simulink model "pidmodel1"  (R2013a)
settings: Solver=ode45  StartTime=0.0  StopTime=10.0  RelTol=1e-3
values from neighbouring files (symbols this model uses):
  A = [0,0,1,0;0,0,0,1;-0,2,3.5,0;0,-3,-2,0]    [at.m]
  B = [0;0;-2;-3]    [at.m]
  C = [1,0,0,0;0,1,0,0;0,0,1,0;0,0,0,1]    [at.m]
  D = [0;0;0;0]    [at.m]
  g = 9.8    [at.m]
  Jp = 0.2    [at.m]
  Jw = 2.3    [at.m]
  Ke = 3    [at.m]
  Kt = 5    [at.m]
  L = 1.8    [at.m]
  mp = 0.9    [at.m]
  mw = 0.2    [at.m]
  n = 0.9    [at.m]
  r = 0.9    [at.m]
  Ra = 0.9    [at.m]
libraries: simulink x2
settings Model: Creator=user  LastModifiedBy=user

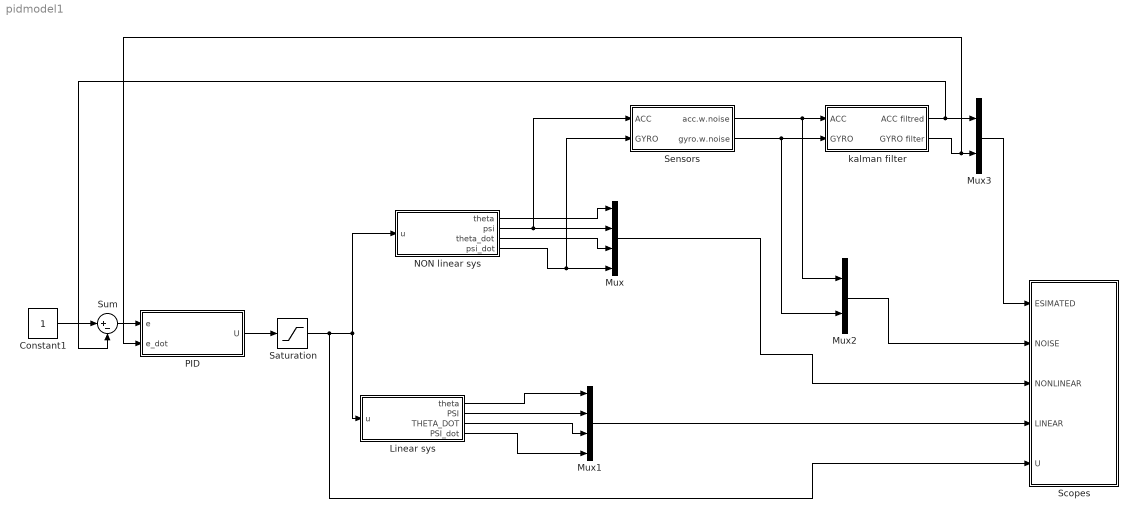
== system pidmodel1 ==
  Constant1 : Constant
  Linear sys : Subsystem
  Mux : Mux
  Mux1 : Mux
  Mux2 : Mux  Inputs=2
  Mux3 : Mux  Inputs=2
  NON linear sys : Subsystem
  "PID " : Subsystem
  Saturation : Saturate
  Scopes : Subsystem
  Sensors : Subsystem
  Sum : Sum  Inputs=|+-
  kalman filter : Subsystem
  wires:
  Sum/1 -> "PID "/1(e)
  Constant1/1 -> Sum/1
  "PID "/1(U) -> Saturation/1
  Linear sys/1(theta) -> Mux1/1
  Linear sys/2(PSI) -> Mux1/2
  Linear sys/3(THETA_DOT) -> Mux1/3
  Linear sys/4(PSI_dot) -> Mux1/4
  NON linear sys/1(theta) -> Mux/1
  NON linear sys/2(psi) -> Sensors/1(ACC), Mux/2
  NON linear sys/3(theta_dot) -> Mux/3
  NON linear sys/4(psi_dot) -> Sensors/2("GYRO "), Mux/4
  Sensors/1(acc.w.noise) -> Mux2/1, kalman filter/1(ACC)
  Sensors/2("gyro.w.noise ") -> Mux2/2, kalman filter/2(GYRO)
  Mux2/1 -> Scopes/2(NOISE)
  Mux3/1 -> Scopes/1(ESIMATED)
  Mux/1 -> Scopes/3(NONLINEAR)
  Mux1/1 -> Scopes/4(LINEAR)
  Saturation/1 -> Scopes/5(U), NON linear sys/1(u), Linear sys/1(u)
  kalman filter/1(ACC filtred) -> Sum/2, Mux3/1
  kalman filter/2(GYRO filter) -> "PID "/2(e_dot), Mux3/2

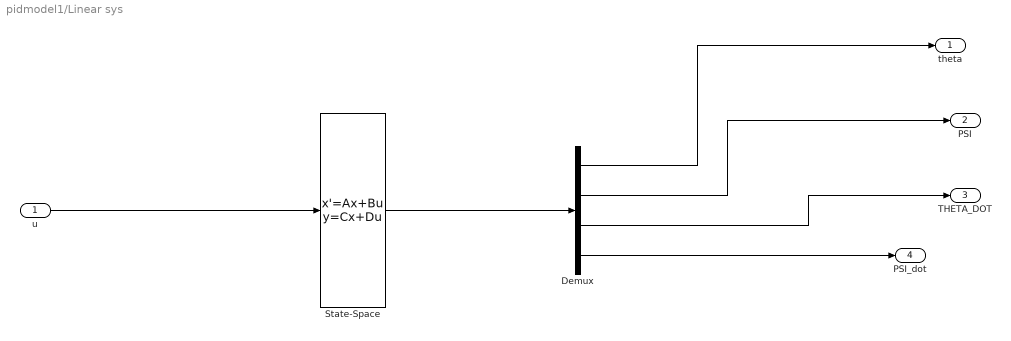
== system pidmodel1/Linear sys ==
  u : Inport
  Demux : Demux
  State-Space : StateSpace  A=A  B=B  C=C  D=D
  theta : Outport
  PSI : Outport  Port=2
  THETA_DOT : Outport  Port=3
  PSI_dot : Outport  Port=4
  wires:
  u/1 -> State-Space/1
  State-Space/1 -> Demux/1
  Demux/1 -> theta/1
  Demux/2 -> PSI/1
  Demux/3 -> THETA_DOT/1
  Demux/4 -> PSI_dot/1

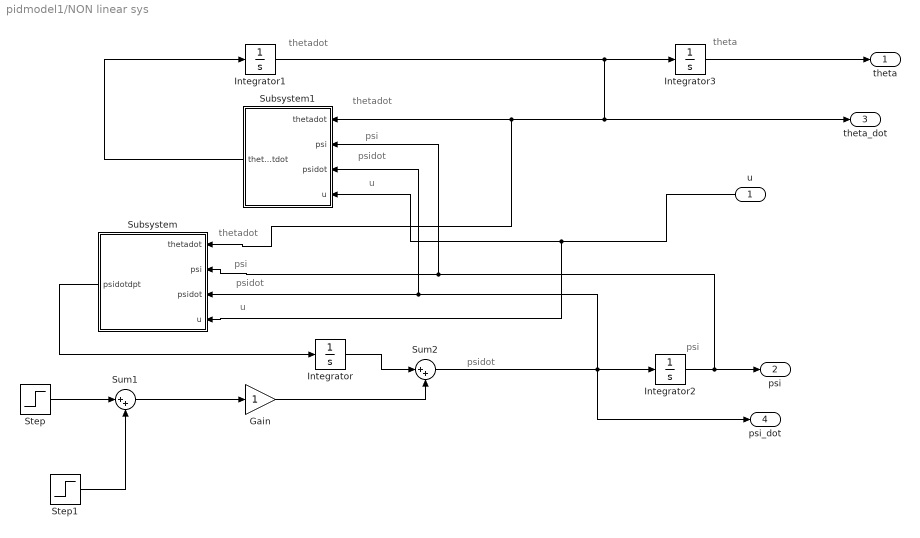
== system pidmodel1/NON linear sys ==
  note: psidot
  note: psi
  note: u
  note: theta
  note: thetadot
  note: psidot
  note: psi
  note: thetadot
  note: u
  note: psidot
  note: psi
  note: thetadot
  u : Inport
  Gain : Gain
  Integrator{,1..3} (4 alike) : Integrator
  Step : Step  SampleTime=0
  Step1 : Step  SampleTime=0
  Subsystem : Subsystem
  Subsystem1 : Subsystem
  Sum1 : Sum  Inputs=|++
  Sum2 : Sum  Inputs=|++
  theta : Outport
  psi : Outport  Port=2
  theta_dot : Outport  Port=3
  psi_dot : Outport  Port=4
  wires:
  Step/1 -> Sum1/1
  Step1/1 -> Sum1/2
  Sum1/1 -> Gain/1
  Gain/1 -> Sum2/2
  Integrator/1 -> Sum2/1
  u/1 -> Subsystem1/4(u), Subsystem/4(u)
  Sum2/1 -> psi_dot/1, Integrator2/1, Subsystem1/3(psidot), Subsystem/3(psidot)
  Integrator2/1 -> Subsystem/2(psi), Subsystem1/2(psi), psi/1
  Integrator1/1 -> Subsystem1/1(thetadot), Subsystem/1(thetadot), theta_dot/1, Integrator3/1
  Integrator3/1 -> theta/1
  Subsystem1/1(thetadotdot) -> Integrator1/1
  Subsystem/1(psidotdpt) -> Integrator/1

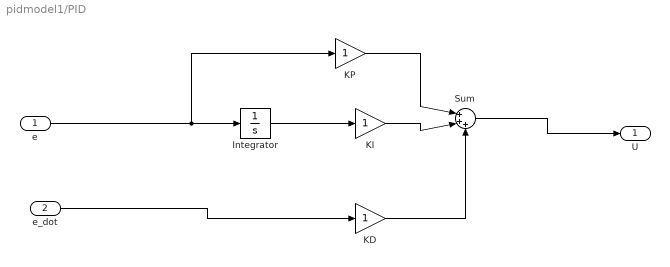
== system pidmodel1/PID  ==
  e : Inport
  e_dot : Inport  Port=2
  Integrator : Integrator
  KD : Gain
  KI : Gain
  KP : Gain
  Sum : Sum  Inputs=|+++
  U : Outport
  wires:
  e/1 -> KP/1, Integrator/1
  Integrator/1 -> KI/1
  e_dot/1 -> KD/1
  Sum/1 -> U/1
  KP/1 -> Sum/1
  KD/1 -> Sum/3
  KI/1 -> Sum/2

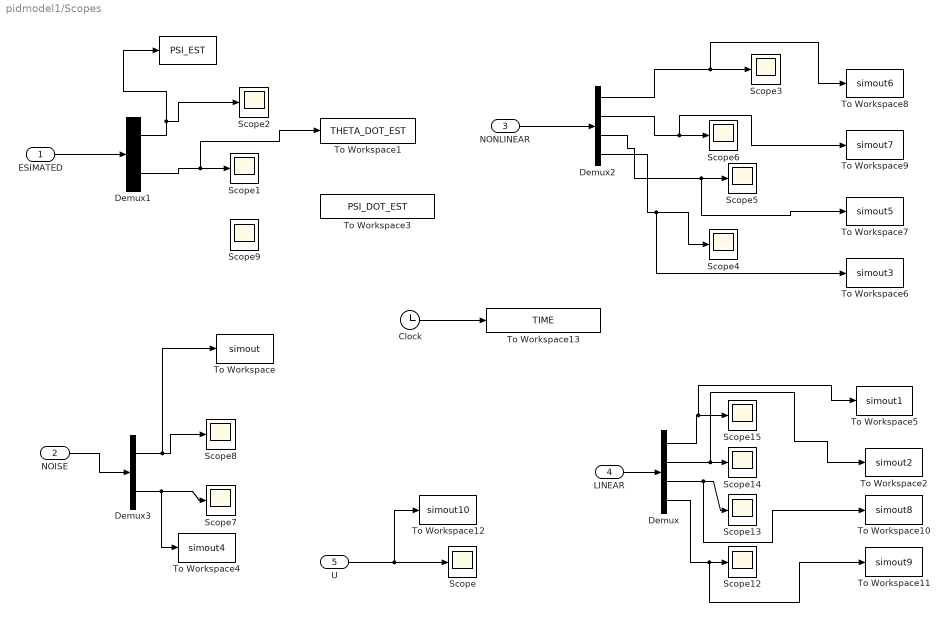
== system pidmodel1/Scopes ==
  ESIMATED : Inport
  NOISE : Inport  Port=2
  NONLINEAR : Inport  Port=3
  LINEAR : Inport  Port=4
  U : Inport  Port=5
  " " : ToWorkspace  VariableName=PSI_EST  SampleTime=-1  SaveFormat=Timeseries
  Clock : Clock
  Demux : Demux
  Demux1 : Demux  Outputs=2
  Demux2 : Demux
  Demux3 : Demux  Outputs=2
  Scope{,1..9,12..15} (14 alike) : Scope
      Scope12 settings: SaveName=ScopeData12
      Scope13 settings: SaveName=ScopeData13
      Scope14 settings: SaveName=ScopeData14
      Scope15 settings: SaveName=ScopeData15
      Scope2 settings: SaveName=ScopeData2
      Scope3 settings: SaveName=ScopeData3
      Scope4 settings: SaveName=ScopeData4
      Scope5 settings: SaveName=ScopeData5
      Scope6 settings: SaveName=ScopeData6
      Scope7 settings: SaveName=ScopeData7
      Scope8 settings: SaveName=ScopeData8
      Scope9 settings: SaveName=ScopeData9
  To Workspace : ToWorkspace  VariableName=simout  SampleTime=-1  SaveFormat=Timeseries
  To Workspace1 : ToWorkspace  VariableName=THETA_DOT_EST  SampleTime=-1  SaveFormat=Timeseries
  To Workspace10 : ToWorkspace  VariableName=simout8  SampleTime=-1  SaveFormat=Timeseries
  To Workspace11 : ToWorkspace  VariableName=simout9  SampleTime=-1  SaveFormat=Timeseries
  To Workspace12 : ToWorkspace  VariableName=simout10  SampleTime=-1  SaveFormat=Timeseries
  To Workspace13 : ToWorkspace  VariableName=TIME  SampleTime=-1  SaveFormat=Timeseries
  To Workspace2 : ToWorkspace  VariableName=simout2  SampleTime=-1  SaveFormat=Timeseries
  To Workspace3 : ToWorkspace  VariableName=PSI_DOT_EST  SampleTime=-1  SaveFormat=Timeseries
  To Workspace4 : ToWorkspace  VariableName=simout4  SampleTime=-1  SaveFormat=Timeseries
  To Workspace5 : ToWorkspace  VariableName=simout1  SampleTime=-1  SaveFormat=Timeseries
  To Workspace6 : ToWorkspace  VariableName=simout3  SampleTime=-1  SaveFormat=Timeseries
  To Workspace7 : ToWorkspace  VariableName=simout5  SampleTime=-1  SaveFormat=Timeseries
  To Workspace8 : ToWorkspace  VariableName=simout6  SampleTime=-1  SaveFormat=Timeseries
  To Workspace9 : ToWorkspace  VariableName=simout7  SampleTime=-1  SaveFormat=Timeseries
  wires:
  ESIMATED/1 -> Demux1/1
  Demux1/1 -> " "/1, Scope2/1
  Demux1/2 -> To Workspace1/1, Scope1/1
  ? -> Scope9/1, To Workspace3/1
  Demux3/2 -> To Workspace4/1, Scope7/1
  Demux3/1 -> To Workspace/1, Scope8/1
  NOISE/1 -> Demux3/1
  NONLINEAR/1 -> Demux2/1
  Demux2/1 -> To Workspace8/1, Scope3/1
  Demux2/2 -> To Workspace9/1, Scope6/1
  Demux2/4 -> To Workspace6/1, Scope4/1
  Demux2/3 -> To Workspace7/1, Scope5/1
  LINEAR/1 -> Demux/1
  Demux/1 -> To Workspace5/1, Scope15/1
  Demux/3 -> To Workspace10/1, Scope13/1
  Demux/2 -> To Workspace2/1, Scope14/1
  Demux/4 -> To Workspace11/1, Scope12/1
  U/1 -> To Workspace12/1, Scope/1
  Clock/1 -> To Workspace13/1

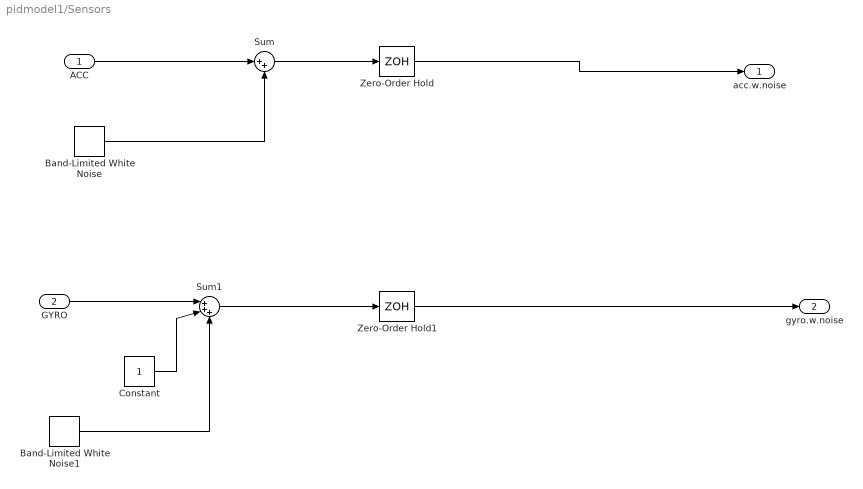
== system pidmodel1/Sensors ==
  ACC : Inport
  "GYRO " : Inport  Port=2
  Band-Limited White Noise : simulink/Sources/Band-Limited White Noise  Cov=[0.1]  Ts=0.1  seed=[23341]
  Band-Limited White Noise1 : simulink/Sources/Band-Limited White Noise  Cov=[0.1]  Ts=0.1  seed=[23341]
  Constant : Constant
  Sum : Sum  Inputs=|++
  Sum1 : Sum  Inputs=|+++
  Zero-Order Hold : ZeroOrderHold
  Zero-Order Hold1 : ZeroOrderHold
  acc.w.noise : Outport
  "gyro.w.noise " : Outport  Port=2
  wires:
  ACC/1 -> Sum/1
  Band-Limited White Noise/1 -> Sum/2
  "GYRO "/1 -> Sum1/1
  Band-Limited White Noise1/1 -> Sum1/3
  Constant/1 -> Sum1/2
  Sum1/1 -> Zero-Order Hold1/1
  Sum/1 -> Zero-Order Hold/1
  Zero-Order Hold/1 -> acc.w.noise/1
  Zero-Order Hold1/1 -> "gyro.w.noise "/1

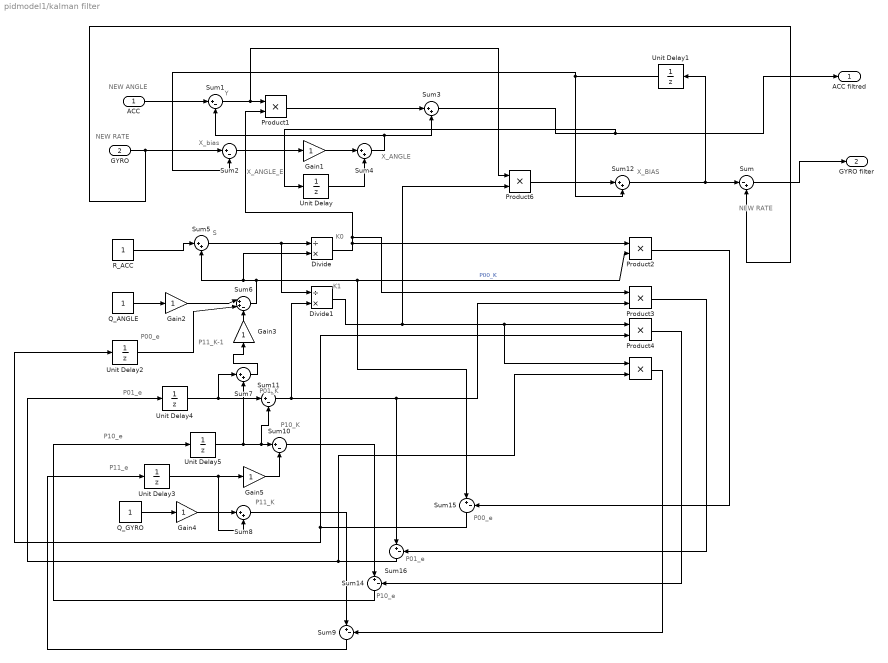
== system pidmodel1/kalman filter ==
  note: NEW RATE
  note: X_BIAS
  note: P10_e
  note: P01_e
  note: P00_e
  note: K1
  note: P01_K
  note: P01_e
  note: P11_e
  note: P10_e
  note: P10_K
  note: P11_K
  note: P00_e
  note: P11_K-1
  note: X_ANGLE_E
  note: X_ANGLE
  note: X_bias
  note: K0
  note: S
  note: Y
  note: NEW RATE
  note: NEW ANGLE
  ACC : Inport
  GYRO : Inport  Port=2
  " " : Product
  Divide : Product  Inputs=/*
  Divide1 : Product  Inputs=/*
  Gain{1..5} (5 alike) : Gain
  Product{1..4,6} (5 alike) : Product
  Q_ANGLE : Constant
  Q_GYRO : Constant
  R_ACC : Constant
  Sum : Sum  Inputs=|-+
  Sum{1..2,9..11,14..16} (8 alike) : Sum  Inputs=|+-
  Sum{3..5,7..8,12} (6 alike) : Sum  Inputs=|++
  Sum6 : Sum  Inputs=|++-
  Unit Delay{,1..5} (6 alike) : UnitDelay  SampleTime=-1
  ACC filtred : Outport
  GYRO filter : Outport  Port=2
  wires:
  ACC/1 -> Sum1/1
  Product1/1 -> Sum3/1
  Sum2/1 -> Gain1/1
  Gain1/1 -> Sum4/1
  Sum4/1 -> Sum3/2, Sum1/2
  R_ACC/1 -> Sum5/1
  Sum5/1 -> Divide1/1, Divide/1
  Q_ANGLE/1 -> Gain2/1
  Gain2/1 -> Sum6/1
  Sum6/1 -> Sum5/2, Divide/2, Sum15/1, Product2/2  "P00_K"
  Gain3/1 -> Sum6/3
  Sum7/1 -> Gain3/1
  Divide/1 -> Product2/1, Product3/1, Product1/2
  Sum3/1 -> Unit Delay/1, ACC filtred/1
  Sum15/1 -> Unit Delay2/1, Product4/2
  Q_GYRO/1 -> Gain4/1
  Gain4/1 -> Sum8/1
  Sum8/1 -> Sum9/1
  " "/1 -> Sum9/2
  Sum9/1 -> Unit Delay3/1
  Unit Delay3/1 -> Gain5/1, Sum8/2
  Gain5/1 -> Sum10/2
  Unit Delay5/1 -> Sum7/2, Sum11/2, Sum10/1
  Sum14/1 -> Unit Delay5/1
  Unit Delay4/1 -> Sum7/1, Sum11/1
  Sum11/1 -> Divide1/2, Sum16/1, Product3/2
  Divide1/1 -> Product6/2, " "/1, Product4/1
  Product2/1 -> Sum15/2
  Product3/1 -> Sum16/2
  Product4/1 -> Sum14/2
  Sum10/1 -> Sum14/1
  Sum16/1 -> " "/2, Unit Delay4/1
  Sum1/1 -> Product6/1, Product1/1
  Product6/1 -> Sum12/1
  Unit Delay1/1 -> Sum2/2, Sum12/2
  Sum12/1 -> Unit Delay1/1, Sum/1
  Sum/1 -> GYRO filter/1
  GYRO/1 -> Sum/2, Sum2/1
  Unit Delay/1 -> Sum4/2
  Unit Delay2/1 -> Sum6/2

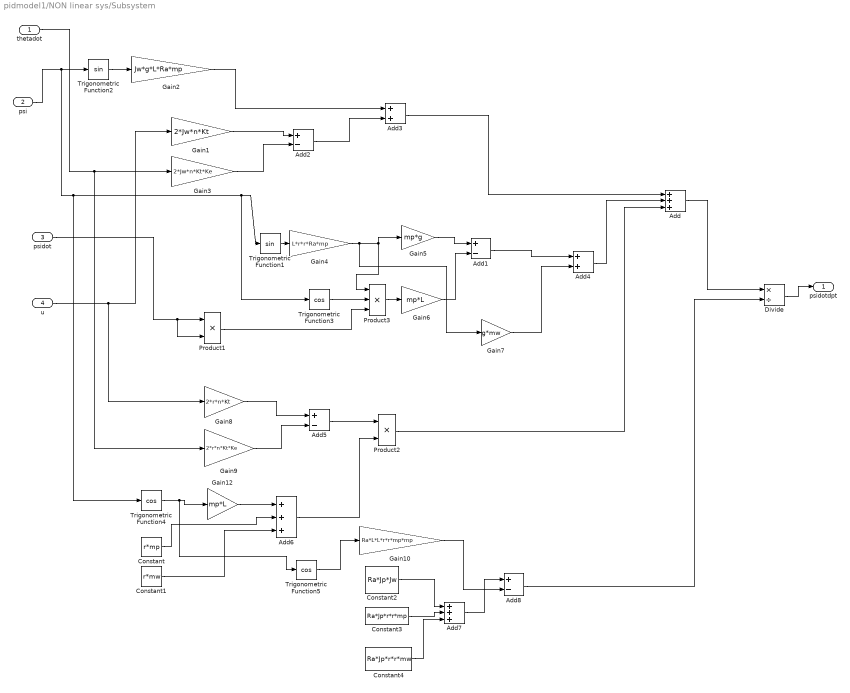
== system pidmodel1/NON linear sys/Subsystem ==
  thetadot : Inport
  psi : Inport  Port=2
  psidot : Inport  Port=3
  u : Inport  Port=4
  Add : Sum  Inputs=+++
  Add{1..2,5,8} (4 alike) : Sum  Inputs=+-
  Add3 : Sum
  Add4 : Sum
  Add6 : Sum  Inputs=+++
  Add7 : Sum  Inputs=+++
  Constant : Constant  Value=r*mp
  Constant1 : Constant  Value=r*mw
  Constant2 : Constant  Value=Ra*Jp*Jw
  Constant3 : Constant  Value=Ra*Jp*r*r*mp
  Constant4 : Constant  Value=Ra*Jp*r*r*mw
  Divide : Product  Inputs=*/
  Gain1 : Gain  Gain=2*Jw*n*Kt
  Gain10 : Gain  Gain=Ra*L*L*r*r*mp*mp
  Gain12 : Gain  Gain=mp*L
  Gain2 : Gain  Gain=Jw*g*L*Ra*mp
  Gain3 : Gain  Gain=2*Jw*n*Kt*Ke
  Gain4 : Gain  Gain=L*r*r*Ra*mp
  Gain5 : Gain  Gain=mp*g
  Gain6 : Gain  Gain=mp*L
  Gain7 : Gain  Gain=g*mw
  Gain8 : Gain  Gain=2*r*n*Kt
  Gain9 : Gain  Gain=2*r*n*Kt*Ke
  Product1 : Product
  Product2 : Product
  Product3 : Product  Inputs=3
  Trigonometric Function1 : Trigonometry
  Trigonometric Function2 : Trigonometry
  Trigonometric Function3 : Trigonometry  Operator=cos
  Trigonometric Function4 : Trigonometry  Operator=cos
  Trigonometric Function5 : Trigonometry  Operator=cos
  psidotdpt : Outport
  wires:
  Gain2/1 -> Add3/1
  u/1 -> Gain8/1, Gain1/1
  Gain1/1 -> Add2/1
  thetadot/1 -> Gain9/1, Gain3/1
  Gain3/1 -> Add2/2
  Add2/1 -> Add3/2
  psi/1 -> Trigonometric Function4/1, Trigonometric Function3/1, Trigonometric Function1/1, Trigonometric Function2/1
  Trigonometric Function2/1 -> Gain2/1
  Add3/1 -> Add/1
  Trigonometric Function1/1 -> Gain4/1
  psidot/1 -> Product1/2, Product1/1
  Gain6/1 -> Add1/2
  Product1/1 -> Product3/3
  Gain5/1 -> Add1/1
  Trigonometric Function3/1 -> Product3/2
  Add1/1 -> Add4/1
  Gain4/1 -> Gain7/1, Product3/1, Gain5/1
  Gain7/1 -> Add4/2
  Add4/1 -> Add/2
  Gain8/1 -> Add5/1
  Gain9/1 -> Add5/2
  Add5/1 -> Product2/1
  Add6/1 -> Product2/2
  Trigonometric Function4/1 -> Gain12/1, Trigonometric Function5/1
  Gain12/1 -> Add6/1
  Constant/1 -> Add6/2
  Constant1/1 -> Add6/3
  Product2/1 -> Add/3
  Add/1 -> Divide/1
  Constant2/1 -> Add7/1
  Constant3/1 -> Add7/2
  Constant4/1 -> Add7/3
  Add7/1 -> Add8/1
  Trigonometric Function5/1 -> Gain10/1
  Gain10/1 -> Add8/2
  Add8/1 -> Divide/2
  Divide/1 -> psidotdpt/1
  Product3/1 -> Gain6/1

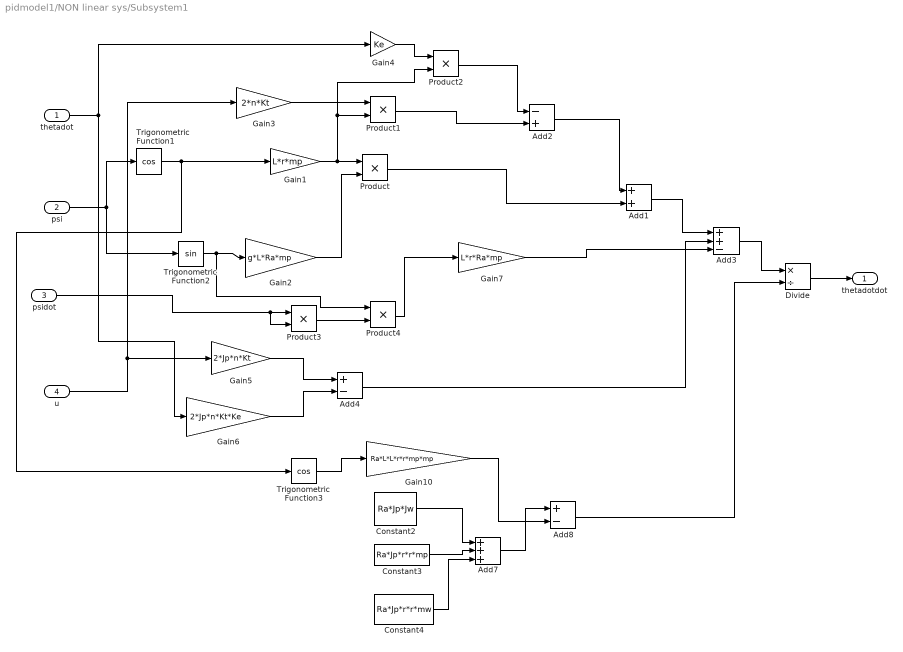
== system pidmodel1/NON linear sys/Subsystem1 ==
  thetadot : Inport
  psi : Inport  Port=2
  psidot : Inport  Port=3
  u : Inport  Port=4
  Add1 : Sum
  Add2 : Sum  Inputs=-+
  Add3 : Sum  Inputs=++-
  Add4 : Sum  Inputs=+-
  Add7 : Sum  Inputs=+++
  Add8 : Sum  Inputs=+-
  Constant2 : Constant  Value=Ra*Jp*Jw
  Constant3 : Constant  Value=Ra*Jp*r*r*mp
  Constant4 : Constant  Value=Ra*Jp*r*r*mw
  Divide : Product  Inputs=*/
  Gain1 : Gain  Gain=L*r*mp
  Gain10 : Gain  Gain=Ra*L*L*r*r*mp*mp
  Gain2 : Gain  Gain=g*L*Ra*mp
  Gain3 : Gain  Gain=2*n*Kt
  Gain4 : Gain  Gain=Ke
  Gain5 : Gain  Gain=2*Jp*n*Kt
  Gain6 : Gain  Gain=2*Jp*n*Kt*Ke
  Gain7 : Gain  Gain=L*r*Ra*mp
  Product{,1..4} (5 alike) : Product
  Trigonometric Function1 : Trigonometry  Operator=cos
  Trigonometric Function2 : Trigonometry
  Trigonometric Function3 : Trigonometry  Operator=cos
  thetadotdot : Outport
  wires:
  Trigonometric Function1/1 -> Trigonometric Function3/1, Gain1/1
  psi/1 -> Trigonometric Function1/1, Trigonometric Function2/1
  Gain1/1 -> Product2/2, Product1/2, Product/1
  Trigonometric Function2/1 -> Product4/1, Gain2/1
  Gain2/1 -> Product/2
  Product/1 -> Add1/2
  u/1 -> Gain3/1, Gain5/1
  Gain3/1 -> Product1/1
  thetadot/1 -> Gain4/1, Gain6/1
  Gain4/1 -> Product2/1
  Product2/1 -> Add2/1
  Add2/1 -> Add1/1
  Add1/1 -> Add3/1
  Add3/1 -> Divide/1
  Divide/1 -> thetadotdot/1
  Gain5/1 -> Add4/1
  Gain6/1 -> Add4/2
  Add4/1 -> Add3/2
  psidot/1 -> Product3/2, Product3/1
  Product3/1 -> Product4/2
  Product1/1 -> Add2/2
  Product4/1 -> Gain7/1
  Gain7/1 -> Add3/3
  Constant2/1 -> Add7/1
  Constant3/1 -> Add7/2
  Constant4/1 -> Add7/3
  Add7/1 -> Add8/1
  Gain10/1 -> Add8/2
  Trigonometric Function3/1 -> Gain10/1
  Add8/1 -> Divide/2
